simulink model "codeGenerationTemplate"  (R2017b)
settings: Solver=FixedStepAuto  StartTime=0.0  StopTime=inf  RelTol=1e-3
PreLoadFcn:
  | % ROS setup
  | rosshutdown;
  | ipAddr = '';
  | rosinit(ipAddr)
  | 
  | % Sample times
  | sampleTime = 0.2;
  | 
  | % Control parameters
  | ctrlParam1 = 2;
  | ctrlParam2 = 3.5;
undefined symbols (not defined in the file): X, Y
libraries: robotlib x3
settings Model: Creator=scastro  LastModifiedBy=scastro
settings OptimizationCC: PassReuseOutputArgsAs=Individual arguments  MaxStackSize=64
settings DebuggingCC: ParameterTunabilityLossMsg=error
settings HardwareCC: ProdBitPerPointer=32  ProdBitPerSizeT=32  ProdBitPerPtrDiffT=32  ProdLargestAtomicFloat=None  ProdIntDivRoundTo=Undefined  ProdEndianess=Unspecified  ProdWordSize=32  ProdHWDeviceType=Generic->Unspecified (assume 32-bit Generic)
settings SFSimCC: MATLABDynamicMemAlloc=off
settings RTWCC: SystemTargetFile=ert.tlc  HardwareBoard=Robot Operating System (ROS)  TemplateMakefile=ert_default_tmf  GenerateReport=on  Toolchain=Catkin  IncludeHyperlinkInReport=on  LaunchReport=on  TargetLang=C++  GenerateTraceInfo=on  GenerateTraceReport=on  GenerateTraceReportSl=on  GenerateTraceReportSf=on  GenerateTraceReportEml=on
settings CodeAppCC: ForceParamTrailComments=on  IgnoreCustomStorageClasses=off  OperatorAnnotations=on  SimulinkDataObjDesc=on  SFDataObjDesc=on  InsertBlockDesc=on

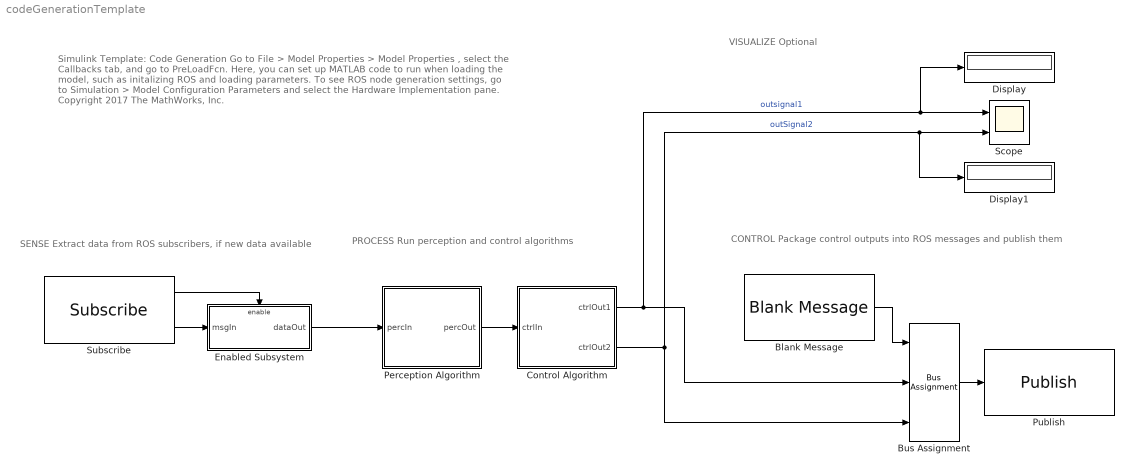
== system codeGenerationTemplate ==
  note: PROCESS
      | Run perception and control algorithms
  note: SENSE
      | Extract data from ROS subscribers, if new data available
  note: VISUALIZE
      | Optional
  note: CONTROL
      | Package control outputs into ROS messages and publish them
  note: Simulink Template: Code Generation
      |
      | Go to File > Model Properties > Model Properties , select the Callbacks tab, and go to PreLoadFcn. Here, you can set up MATLAB code to run when loading the model, such as initalizing ROS and loading parameters.
      |
      | To see ROS node generation settings, go to Simulation > Model Configuration Parameters and select the Hardware Implementation pane.
      |
      | Copyright 2017 The MathWorks, Inc.
  Blank Message : robotlib/Blank Message  SourceLibraryInfo=This block requires Robotics System Toolbox  messageType=geometry_msgs/Point  SampleTime=inf
      settings: SourceProductBaseCode=RO
  Bus Assignment : BusAssignment  AssignedSignals=X,Y
  Control Algorithm : Subsystem
  Display : Display
  Display1 : Display
  Enabled Subsystem : Subsystem  TreatAsAtomicUnit=on
  Perception Algorithm : Subsystem
  Publish : robotlib/Publish  SourceLibraryInfo=This block requires Robotics System Toolbox  topicSource=Specify your own  topic=/my_pub_topic  messageType=geometry_msgs/Point  messageQueueLength=1
      settings: SourceProductBaseCode=RO
  Scope : Scope  NumInputPorts=2
  Subscribe : robotlib/Subscribe  SourceLibraryInfo=This block requires Robotics System Toolbox  topicSource=Select from ROS network  topic=/my_sub_topic  messageType=geometry_msgs/Point  sampleTime=-1  messageQueueLength=1
      settings: SourceProductBaseCode=RO
  wires:
  Enabled Subsystem/1(dataOut) -> Perception Algorithm/1(percIn)
  Subscribe/2 -> Enabled Subsystem/1(msgIn)
  Subscribe/1 -> Enabled Subsystem/Enable
  Bus Assignment/1 -> Publish/1
  Blank Message/1 -> Bus Assignment/1
  Control Algorithm/1(ctrlOut1) -> Bus Assignment/2, Display/1, Scope/1  "outsignal1"
  Control Algorithm/2(ctrlOut2) -> Display1/1, Scope/2, Bus Assignment/3  "outSignal2"
  Perception Algorithm/1(percOut) -> Control Algorithm/1(ctrlIn)

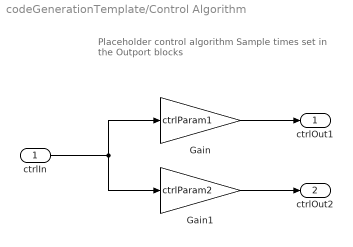
== system codeGenerationTemplate/Control Algorithm ==
  note: Placeholder control algorithm
      |
      | Sample times set in the Outport blocks
  ctrlIn : Inport
  Gain : Gain  Gain=ctrlParam1
  Gain1 : Gain  Gain=ctrlParam2
  ctrlOut1 : Outport  SampleTime=sampleTime
      settings: AttributesFormatString=Sample time: %<SampleTime>
  ctrlOut2 : Outport  Port=2  SampleTime=sampleTime
      settings: AttributesFormatString=Sample time: %<SampleTime>
  wires:
  ctrlIn/1 -> Gain1/1, Gain/1
  Gain/1 -> ctrlOut1/1
  Gain1/1 -> ctrlOut2/1

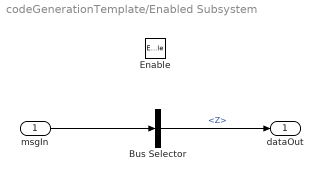
== system codeGenerationTemplate/Enabled Subsystem ==
  msgIn : Inport
  Enable : EnablePort
  Bus Selector : BusSelector  OutputSignals=Z
  dataOut : Outport
  wires:
  msgIn/1 -> Bus Selector/1
  Bus Selector/1 -> dataOut/1  "<Z>"

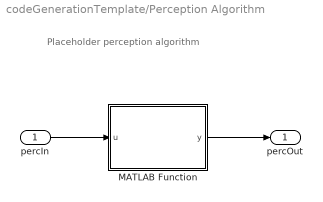
== system codeGenerationTemplate/Perception Algorithm ==
  note: Placeholder perception algorithm
  percIn : Inport
  MATLAB Function : MATLAB Function  TreatAsAtomicUnit=on
  percOut : Outport
  wires:
  percIn/1 -> MATLAB Function/1(u)
  MATLAB Function/1(y) -> percOut/1

== matlab function codeGenerationTemplate/Perception Algorithm/MATLAB Function ==
  data: u input; y output
function y = myPerceptionFcn(u)

y = 2*u;
